simulink model "Fan_DD"  (R2016b)
settings: configuration reference "CodeGenConfigSet" (kept outside this file)
values from neighbouring files (symbols this model uses):
  DTY_CYC_MIN = fi(0,DutyCycle_rate)    [init_Fan_DD.m]
  Fan_PwmOut2_rMax_C = Calibration.Parameter    [init_Fan_DD.m]
  Fan_PwmOut2_rMin_C = Calibration.Parameter    [init_Fan_DD.m]
  Fan_PwmOut2_swtBattCor_C = Calibration.Parameter    [init_Fan_DD.m]
  Fan_PwmOut_rMax_C = Calibration.Parameter    [init_Fan_DD.m]
  Fan_PwmOut_rMin_C = Calibration.Parameter    [init_Fan_DD.m]
  Fan_PwmOut_swtBattCor_C = Calibration.Parameter    [init_Fan_DD.m]
  Fan_rCnv2_CUR = Calibration.Parameter    [init_Fan_DD.m]
  Fan_rCnv2_CURX = Calibration.Parameter    [init_Fan_DD.m]
  Fan_rCnv_CUR = Calibration.Parameter    [init_Fan_DD.m]
  Fan_rCnv_CURX = Calibration.Parameter    [init_Fan_DD.m]
  Fan_rPsDisbl2_C = Calibration.Parameter    [init_Fan_DD.m]
  Fan_rPsDisbl_C = Calibration.Parameter    [init_Fan_DD.m]
  Fan_stPsDiaDisblPWM2_C = Calibration.Parameter    [init_Fan_DD.m]
  Fan_stPsDiaDisblPWM_C = Calibration.Parameter    [init_Fan_DD.m]
  Fan_stPsDisblPWM2_C = Calibration.Parameter    [init_Fan_DD.m]
  Fan_stPsDisblPWM_C = Calibration.Parameter    [init_Fan_DD.m]
  Fan_stPsDisDIO2_C = Calibration.Parameter    [init_Fan_DD.m]
  Fan_stPsDisDIO_C = Calibration.Parameter    [init_Fan_DD.m]
  Fan_swtSYDia2_C = Calibration.Parameter    [init_Fan_DD.m]
  Fan_swtSYDia_C = Calibration.Parameter    [init_Fan_DD.m]
  Fan_tiFanCyc_C = Calibration.Parameter    [init_Fan_DD.m]
libraries: simulink x6, CXLib x2
settings Model: Creator=xinchangran  LastModifiedBy=xinchangran
settings ConfigSetRef: SourceLocation=Base Workspace

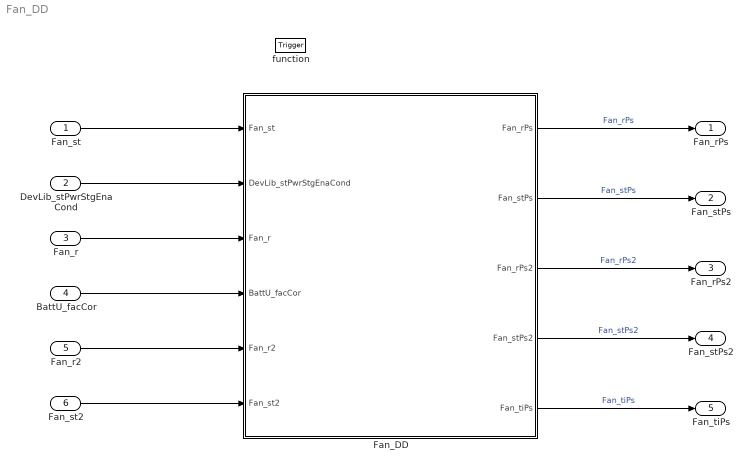
== system Fan_DD ==
  Fan_st : Inport  OutMin=0  OutMax=1  OutDataTypeStr=boolean
  DevLib_stPwrStgEnaCond : Inport  Description=Control unit status relevant to power stage deactivation/error diagnosis  Port=2  OutMin=0  OutMax=65535  OutDataTypeStr=State_uint16
  Fan_r : Inport  Tag=%  Description=Actuator setpoint value for the first fan output  Port=3  OutMin=0  OutMax=100  OutDataTypeStr=DutyCycle_rate
  BattU_facCor : Inport  Description=Battery correction factor  Port=4  OutMin=-32  OutMax=31.9  OutDataTypeStr=Factor
  Fan_r2 : Inport  Tag=%  Description=set point duty cycle for PWM fan power stage 2  Port=5  OutMin=0  OutMax=100  OutDataTypeStr=DutyCycle_rate
  Fan_st2 : Inport  Description=Fan 2 status based on fan opening  Port=6  OutMin=0  OutMax=1  OutDataTypeStr=boolean
  function : TriggerPort  TriggerType=function-call  VariantControl=Variant
  Fan_DD : Subsystem
  Fan_rPs : Outport  Tag=%  Description=Fan duty cycle  OutMin=0  OutMax=100  OutDataTypeStr=DutyCycle_rate
  Fan_stPs : Outport  Description=fan output state  Port=2  OutMin=0  OutMax=1  OutDataTypeStr=boolean
  Fan_rPs2 : Outport  Tag=%  Description=Fan 2 duty cycle  Port=3  OutMin=0  OutMax=100  OutDataTypeStr=DutyCycle_rate
  Fan_stPs2 : Outport  Description=fan 2 output state  Port=4  OutMin=0  OutMax=1  OutDataTypeStr=boolean
  Fan_tiPs : Outport  Tag=ms  Description=fan cycle  Port=5  OutMin=0  OutMax=65535  OutDataTypeStr=Debounce_ms
  wires:
  Fan_st/1 -> Fan_DD/1(Fan_st)
  DevLib_stPwrStgEnaCond/1 -> Fan_DD/2(DevLib_stPwrStgEnaCond)
  Fan_r/1 -> Fan_DD/3(Fan_r)
  BattU_facCor/1 -> Fan_DD/4(BattU_facCor)
  Fan_r2/1 -> Fan_DD/5(Fan_r2)
  Fan_st2/1 -> Fan_DD/6(Fan_st2)
  Fan_DD/1(Fan_rPs) -> Fan_rPs/1  "Fan_rPs"
  Fan_DD/2(Fan_stPs) -> Fan_stPs/1  "Fan_stPs"
  Fan_DD/3(Fan_rPs2) -> Fan_rPs2/1  "Fan_rPs2"
  Fan_DD/4(Fan_stPs2) -> Fan_stPs2/1  "Fan_stPs2"
  Fan_DD/5(Fan_tiPs) -> Fan_tiPs/1  "Fan_tiPs"

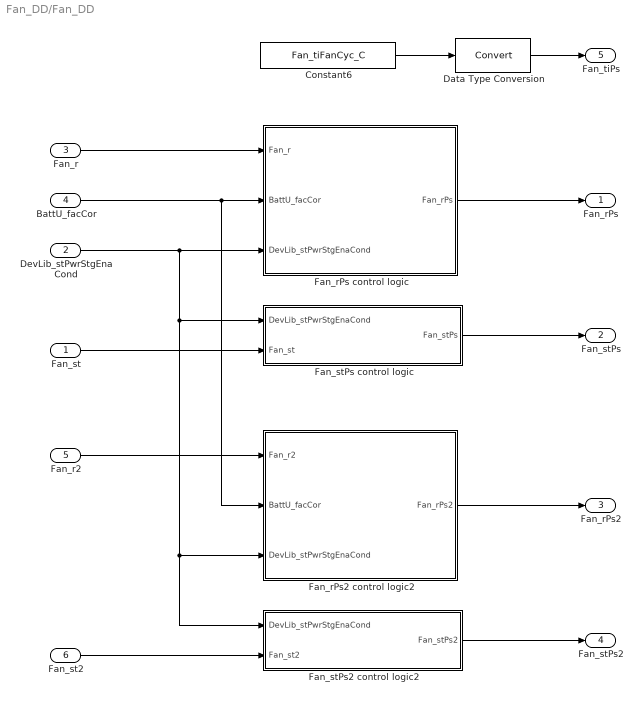
== system Fan_DD/Fan_DD ==
  Fan_st : Inport  OutMin=0  OutMax=1  OutDataTypeStr=boolean
  DevLib_stPwrStgEnaCond : Inport  Description=Control unit status relevant to power stage deactivation/error diagnosis  Port=2  OutMin=0  OutMax=65535  OutDataTypeStr=State_uint16
  Fan_r : Inport  Tag=%  Description=Actuator setpoint value for the first fan output  Port=3  OutMin=0  OutMax=100  OutDataTypeStr=DutyCycle_rate
  BattU_facCor : Inport  Description=Battery correction factor  Port=4  OutMin=-32  OutMax=31.9  OutDataTypeStr=Factor
  Fan_r2 : Inport  Tag=%  Description=set point duty cycle for PWM fan power stage 2  Port=5  OutMin=0  OutMax=100  OutDataTypeStr=DutyCycle_rate
  Fan_st2 : Inport  Description=Fan 2 status based on fan opening  Port=6  OutMin=0  OutMax=1  OutDataTypeStr=boolean
  Constant6 : Constant  Value=Fan_tiFanCyc_C
  Data Type Conversion : DataTypeConversion
  Fan_rPs control logic : Subsystem
  Fan_rPs2 control logic2 : Subsystem
  Fan_stPs control logic : Subsystem
  Fan_stPs2 control logic2 : Subsystem
  Fan_rPs : Outport  Tag=%  Description=Fan duty cycle  OutMin=0  OutMax=100  OutDataTypeStr=DutyCycle_rate
  Fan_stPs : Outport  Description=fan output state  Port=2  OutMin=0  OutMax=1  OutDataTypeStr=boolean
  Fan_rPs2 : Outport  Tag=%  Description=Fan 2 duty cycle  Port=3  OutMin=0  OutMax=100  OutDataTypeStr=DutyCycle_rate
  Fan_stPs2 : Outport  Description=fan 2 output state  Port=4  OutMin=0  OutMax=1  OutDataTypeStr=boolean
  Fan_tiPs : Outport  Tag=ms  Description=fan cycle  Port=5  OutMin=0  OutMax=65535  OutDataTypeStr=Debounce_ms
  wires:
  Fan_r/1 -> Fan_rPs control logic/1(Fan_r)
  Fan_rPs control logic/1(Fan_rPs) -> Fan_rPs/1
  Fan_st/1 -> Fan_stPs control logic/2(Fan_st)
  Fan_stPs control logic/1(Fan_stPs) -> Fan_stPs/1
  Fan_r2/1 -> Fan_rPs2 control logic2/1(Fan_r2)
  Constant6/1 -> Data Type Conversion/1
  Data Type Conversion/1 -> Fan_tiPs/1
  Fan_st2/1 -> Fan_stPs2 control logic2/2(Fan_st2)
  DevLib_stPwrStgEnaCond/1 -> Fan_rPs control logic/3(DevLib_stPwrStgEnaCond), Fan_stPs2 control logic2/1(DevLib_stPwrStgEnaCond), Fan_rPs2 control logic2/3(DevLib_stPwrStgEnaCond), Fan_stPs control logic/1(DevLib_stPwrStgEnaCond)
  Fan_stPs2 control logic2/1(Fan_stPs2) -> Fan_stPs2/1
  BattU_facCor/1 -> Fan_rPs2 control logic2/2(BattU_facCor), Fan_rPs control logic/2(BattU_facCor)
  Fan_rPs2 control logic2/1(Fan_rPs2) -> Fan_rPs2/1

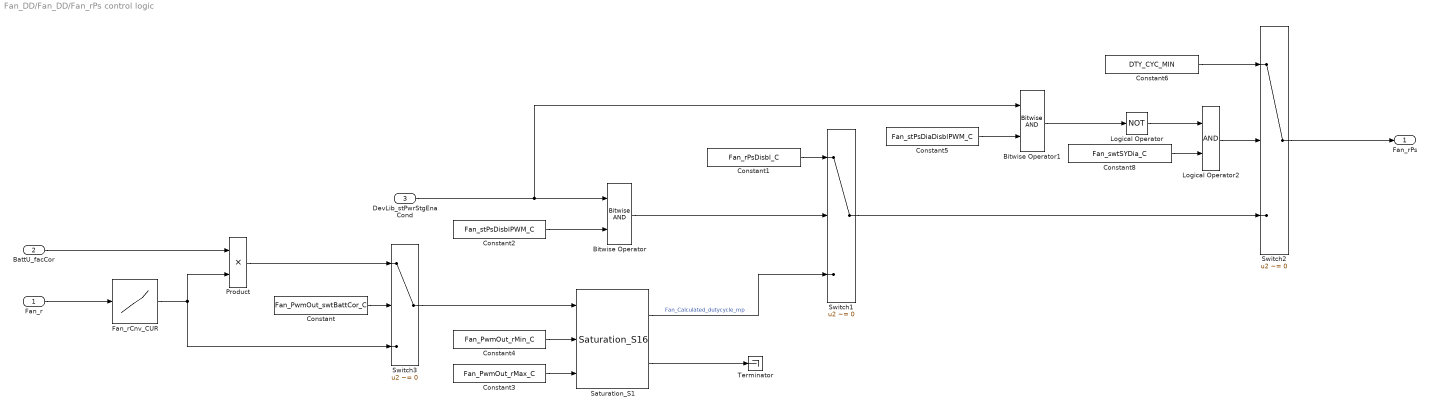
== system Fan_DD/Fan_DD/Fan_rPs control logic ==
  Fan_r : Inport  Tag=%  OutMin=0  OutMax=100  OutDataTypeStr=DutyCycle_rate
  BattU_facCor : Inport  Description=Battery correction factor  Port=2  OutMin=-32  OutMax=31.9
  DevLib_stPwrStgEnaCond : Inport  Description=Control unit status relevant to power stage deactivation/error diagnosis  Port=3  OutMin=0  OutMax=65535
  Bitwise Operator : simulink/Logic and Bit Operations/Bitwise Operator  logicop=AND  UseBitMask=off  NumInputPorts=2  BitMask=bin2dec('11011001')  BitMaskRealWorld=Stored Integer
  Bitwise Operator1 : simulink/Logic and Bit Operations/Bitwise Operator  logicop=AND  UseBitMask=off  NumInputPorts=2  BitMask=bin2dec('11011001')  BitMaskRealWorld=Stored Integer
  Constant : Constant  Value=Fan_PwmOut_swtBattCor_C
  Constant1 : Constant  Value=Fan_rPsDisbl_C
  Constant2 : Constant  Value=Fan_stPsDisblPWM_C
  Constant3 : Constant  Value=Fan_PwmOut_rMax_C
  Constant4 : Constant  Value=Fan_PwmOut_rMin_C
  Constant5 : Constant  Value=Fan_stPsDiaDisblPWM_C
  Constant6 : Constant  Value=DTY_CYC_MIN
  Constant8 : Constant  Value=Fan_swtSYDia_C
  Fan_rCnv_CUR : Lookup_n-D  NumberOfTableDimensions=1  BreakpointsForDimension1=Fan_rCnv_CURX  BreakpointsForDimension1DataTypeStr=Inherit: Inherit from 'Breakpoint data'  BeginIndexSearchUsingPreviousIndexResult=on  Table=Fan_rCnv_CUR  ExtrapMethod=Clip  UseLastTableValue=on  InternalRulePriority=Speed  OutDataTypeStr=Inherit: Inherit from 'Table data'  RndMeth=Simplest  SaturateOnIntegerOverflow=on
  Logical Operator : Logic  Operator=NOT  AllPortsSameDT=off  OutDataTypeStr=boolean
  Logical Operator2 : Logic  AllPortsSameDT=off  OutDataTypeStr=boolean
  Product : Product  OutDataTypeStr=Inherit: Inherit via back propagation  SaturateOnIntegerOverflow=on
  Saturation_S1 : CXLib/Saturation_S16
  Switch1 : Switch  Criteria=u2 ~= 0  SaturateOnIntegerOverflow=on  InputSameDT=on
  Switch2 : Switch  Criteria=u2 ~= 0  SaturateOnIntegerOverflow=on  InputSameDT=on
  Switch3 : Switch  Criteria=u2 ~= 0  SaturateOnIntegerOverflow=on  InputSameDT=on
  Terminator : Terminator
  Fan_rPs : Outport  Tag=%  Description=Fan duty cycle  OutMin=0  OutMax=100  OutDataTypeStr=DutyCycle_rate
  wires:
  Constant6/1 -> Switch2/1
  Constant2/1 -> Bitwise Operator/2
  Switch3/1 -> Saturation_S1/1
  Product/1 -> Switch3/1
  Fan_rCnv_CUR/1 -> Switch3/3, Product/2
  Constant1/1 -> Switch1/1
  BattU_facCor/1 -> Product/1
  Fan_r/1 -> Fan_rCnv_CUR/1
  Switch1/1 -> Switch2/3
  Switch2/1 -> Fan_rPs/1
  Saturation_S1/2 -> Terminator/1
  Constant5/1 -> Bitwise Operator1/2
  Bitwise Operator1/1 -> Logical Operator/1
  Saturation_S1/1 -> Switch1/3  "Fan_Calculated_dutycycle_mp"
  Constant/1 -> Switch3/2
  Constant3/1 -> Saturation_S1/3
  Constant4/1 -> Saturation_S1/2
  Bitwise Operator/1 -> Switch1/2
  Constant8/1 -> Logical Operator2/2
  Logical Operator/1 -> Logical Operator2/1
  Logical Operator2/1 -> Switch2/2
  DevLib_stPwrStgEnaCond/1 -> Bitwise Operator1/1, Bitwise Operator/1

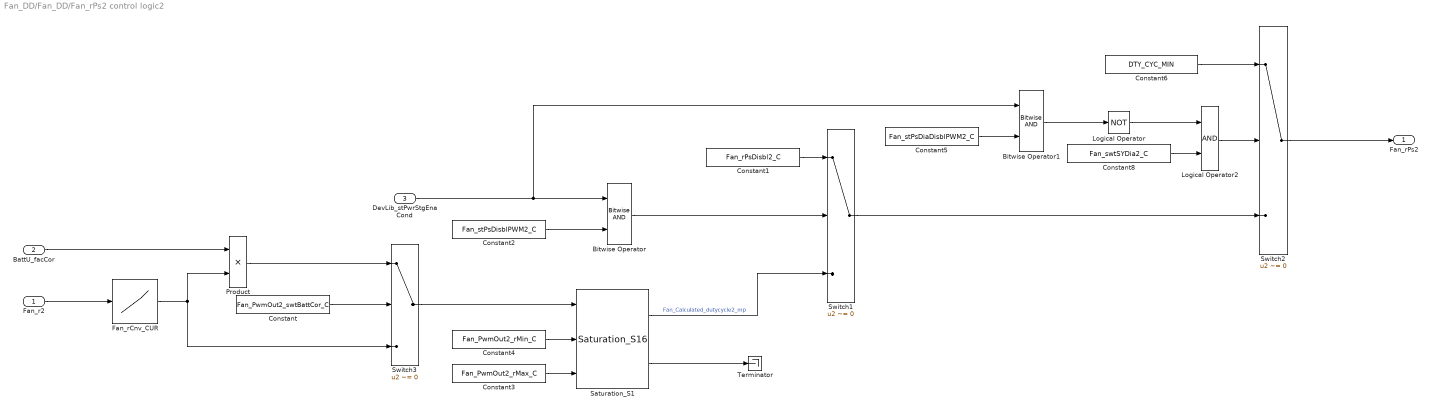
== system Fan_DD/Fan_DD/Fan_rPs2 control logic2 ==
  Fan_r2 : Inport  Tag=%  OutMin=0  OutMax=100  OutDataTypeStr=DutyCycle_rate
  BattU_facCor : Inport  Description=Battery correction factor  Port=2  OutMin=-32  OutMax=31.9
  DevLib_stPwrStgEnaCond : Inport  Description=Control unit status relevant to power stage deactivation/error diagnosis  Port=3  OutMin=0  OutMax=65535
  Bitwise Operator : simulink/Logic and Bit Operations/Bitwise Operator  logicop=AND  UseBitMask=off  NumInputPorts=2  BitMask=bin2dec('11011001')  BitMaskRealWorld=Stored Integer
  Bitwise Operator1 : simulink/Logic and Bit Operations/Bitwise Operator  logicop=AND  UseBitMask=off  NumInputPorts=2  BitMask=bin2dec('11011001')  BitMaskRealWorld=Stored Integer
  Constant : Constant  Value=Fan_PwmOut2_swtBattCor_C
  Constant1 : Constant  Value=Fan_rPsDisbl2_C
  Constant2 : Constant  Value=Fan_stPsDisblPWM2_C
  Constant3 : Constant  Value=Fan_PwmOut2_rMax_C
  Constant4 : Constant  Value=Fan_PwmOut2_rMin_C
  Constant5 : Constant  Value=Fan_stPsDiaDisblPWM2_C
  Constant6 : Constant  Value=DTY_CYC_MIN
  Constant8 : Constant  Value=Fan_swtSYDia2_C
  Fan_rCnv_CUR : Lookup_n-D  NumberOfTableDimensions=1  BreakpointsForDimension1=Fan_rCnv2_CURX  BreakpointsForDimension1DataTypeStr=Inherit: Inherit from 'Breakpoint data'  BeginIndexSearchUsingPreviousIndexResult=on  Table=Fan_rCnv2_CUR  ExtrapMethod=Clip  UseLastTableValue=on  InternalRulePriority=Speed  OutDataTypeStr=Inherit: Inherit from 'Table data'  RndMeth=Simplest  SaturateOnIntegerOverflow=on
  Logical Operator : Logic  Operator=NOT  AllPortsSameDT=off  OutDataTypeStr=boolean
  Logical Operator2 : Logic  AllPortsSameDT=off  OutDataTypeStr=boolean
  Product : Product  OutDataTypeStr=Inherit: Inherit via back propagation  SaturateOnIntegerOverflow=on
  Saturation_S1 : CXLib/Saturation_S16
  Switch1 : Switch  Criteria=u2 ~= 0  SaturateOnIntegerOverflow=on  InputSameDT=on
  Switch2 : Switch  Criteria=u2 ~= 0  SaturateOnIntegerOverflow=on  InputSameDT=on
  Switch3 : Switch  Criteria=u2 ~= 0  SaturateOnIntegerOverflow=on  InputSameDT=on
  Terminator : Terminator
  Fan_rPs2 : Outport  Tag=%  Description=Fan duty cycle  OutMin=0  OutMax=100  OutDataTypeStr=DutyCycle_rate
  wires:
  DevLib_stPwrStgEnaCond/1 -> Bitwise Operator/1, Bitwise Operator1/1
  Logical Operator2/1 -> Switch2/2
  Logical Operator/1 -> Logical Operator2/1
  Constant8/1 -> Logical Operator2/2
  Bitwise Operator/1 -> Switch1/2
  Constant4/1 -> Saturation_S1/2
  Constant3/1 -> Saturation_S1/3
  Constant/1 -> Switch3/2
  Saturation_S1/1 -> Switch1/3  "Fan_Calculated_dutycycle2_mp"
  Bitwise Operator1/1 -> Logical Operator/1
  Constant5/1 -> Bitwise Operator1/2
  Saturation_S1/2 -> Terminator/1
  Switch2/1 -> Fan_rPs2/1
  Switch1/1 -> Switch2/3
  Fan_r2/1 -> Fan_rCnv_CUR/1
  BattU_facCor/1 -> Product/1
  Constant1/1 -> Switch1/1
  Fan_rCnv_CUR/1 -> Product/2, Switch3/3
  Product/1 -> Switch3/1
  Switch3/1 -> Saturation_S1/1
  Constant2/1 -> Bitwise Operator/2
  Constant6/1 -> Switch2/1

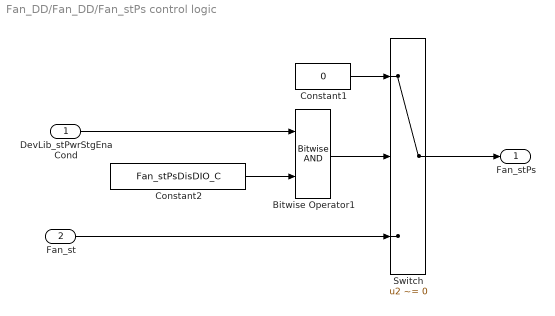
== system Fan_DD/Fan_DD/Fan_stPs control logic ==
  DevLib_stPwrStgEnaCond : Inport
  Fan_st : Inport  Port=2  OutMin=0  OutMax=1
  Bitwise Operator1 : simulink/Logic and Bit Operations/Bitwise Operator  logicop=AND  UseBitMask=off  NumInputPorts=2  BitMask=bin2dec('11011001')  BitMaskRealWorld=Stored Integer
  Constant1 : Constant  Value=0  OutDataTypeStr=Inherit: Inherit via back propagation
  Constant2 : Constant  Value=Fan_stPsDisDIO_C
  Switch : Switch  Criteria=u2 ~= 0  InputSameDT=on
  Fan_stPs : Outport  Description=fan output state  OutMin=0  OutMax=1  OutDataTypeStr=boolean
  wires:
  Bitwise Operator1/1 -> Switch/2
  Constant1/1 -> Switch/1
  Fan_st/1 -> Switch/3
  Switch/1 -> Fan_stPs/1
  Constant2/1 -> Bitwise Operator1/2
  DevLib_stPwrStgEnaCond/1 -> Bitwise Operator1/1

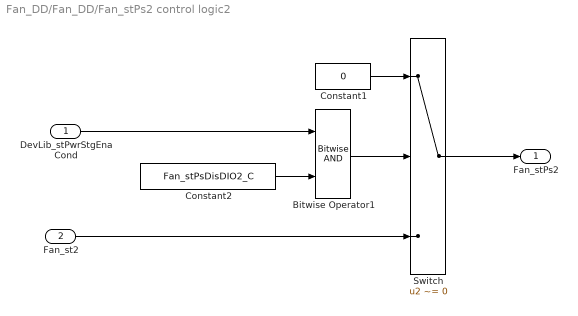
== system Fan_DD/Fan_DD/Fan_stPs2 control logic2 ==
  DevLib_stPwrStgEnaCond : Inport
  Fan_st2 : Inport  Port=2  OutMin=0  OutMax=1
  Bitwise Operator1 : simulink/Logic and Bit Operations/Bitwise Operator  logicop=AND  UseBitMask=off  NumInputPorts=2  BitMask=bin2dec('11011001')  BitMaskRealWorld=Stored Integer
  Constant1 : Constant  Value=0  OutDataTypeStr=Inherit: Inherit via back propagation
  Constant2 : Constant  Value=Fan_stPsDisDIO2_C
  Switch : Switch  Criteria=u2 ~= 0  InputSameDT=on
  Fan_stPs2 : Outport  Description=fan output state  OutMin=0  OutMax=1  OutDataTypeStr=boolean
  wires:
  DevLib_stPwrStgEnaCond/1 -> Bitwise Operator1/1
  Constant2/1 -> Bitwise Operator1/2
  Switch/1 -> Fan_stPs2/1
  Fan_st2/1 -> Switch/3
  Constant1/1 -> Switch/1
  Bitwise Operator1/1 -> Switch/2
